simulink model "EDF2Tareas"  (R2021b)
settings: Solver=VariableStepAuto  StartTime=0.0  StopTime=0.2  RelTol=1e-3
values from neighbouring files (symbols this model uses):
  a = [8.878e-12  1.776e-11   2.663e-11]/0.0274    [GeneracionDatos.m]
  b = [1.291e-5   2.583e-5    3.874e-5]/0.0274    [GeneracionDatos.m]
  c = 0.0007648*[1 1 1]/0.0274    [GeneracionDatos.m]    (also in planner.m = zeros(N, 1))
  D = 0*[1 1 1]    [GeneracionDatos.m]
  H = H*gran    (= 0.001)    [GeneracionDatos.m]
  I = [5.1249     3.1462   1.4256]    [GeneracionDatos.m]
  N = length(h)    [GeneracionDatos.m]
  P = [0.028842   0.035017 0.039862]    [GeneracionDatos.m]
undefined symbols (not defined in the file or in its folder): m
libraries: slpidlib x3, sldelib x1
settings Model: Creator=YayoCG  LastModifiedBy=mluser
settings SolverCC: AlgebraicLoopSolver=TrustRegion
settings DebuggingCC: SFMachineParentedDataDiag=warning

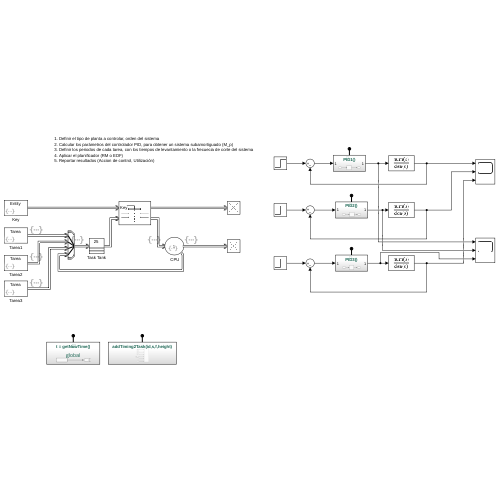
[thumbnail: Simulink's stored preview of the top-level diagram]
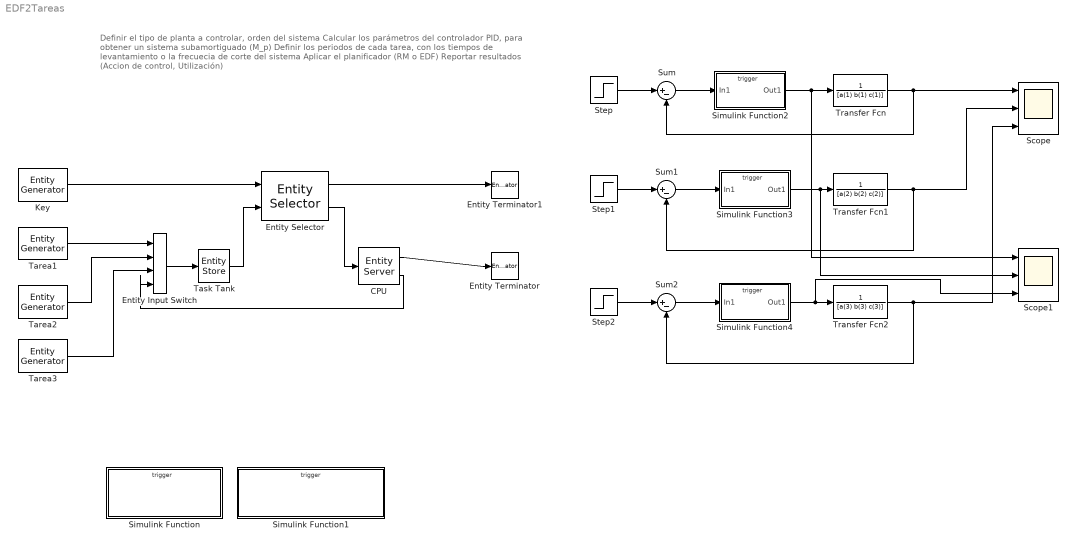
== system EDF2Tareas ==
  note: Definir el tipo de planta a controlar, orden del sistema
      | Calcular los parámetros del controlador PID, para obtener un sistema subamortiguado (M_p)
      | Definir los periodos de cada tarea, con los tiempos de levantamiento o la frecuecia de corte del sistema
      | Aplicar el planificador (RM o EDF)
      | Reportar resultados (Accion de control, Utilización)
  " CPU" : EntityServer  InputPortMessageModes=m  OutputPortMessageModes=m,m  Capacity=1  ServiceTimeSource=Attribute  ServiceTimeAttributeName=C  ServiceTimeAction=dt = entity.C + 0*rand(1,1);  EntryAction=|  ExitAction=|  PreemptAction=|  PermitPreemptionBasedOnAttribute=on  SortingAttributeName=C  WriteResidualTimeToAttribute=on  ResidualTimeAttributeName=C
      EntryAction=|
      | entity.priority = 2;
      | s = getNowTime();
      | entity.s = s;
      ExitAction=|
      | f = getNowTime();
      | addTiming2Task(entity.id, entity.s, f, 0.5);
      | 
      | switch entity.id
      |     case 1
      |         PID1();
      |     case 2
      |         PID2();
      |     case 3
      |         PID3();
      | end
      PreemptAction=|
      | %
      | f = getNowTime();
      | addTiming2Task(entity.id, entity.s, f, 0.5);
      settings: OutputPortMap=o9,o10
  Entity Input Switch : EntityInputSwitch  InputPortMessageModes=m,m,m,m  OutputPortMessageModes=m  NumberInputPorts=4
      settings: InputPortMap=u1,u2,u3,u4
  Entity Selector : sldelib/Entity Selector  mNumberOfStreams=1  mKeyEntityAttributeName={'key'}  mEntityAttributeName={'id'}  mMatchingNumberSource=Dialog  mNumberOfMatches=1  mNumberOfMatchesAttribute=Name  mNumEntitiesDepOpt=off  mNumEntitiesInBlockOpt=off  mNumEntitiesExtractedOpt=off
      settings: SourceProductBaseCode=SE
  Entity Terminator : EntityTerminator  InputPortMessageModes=m
  Entity Terminator1 : EntityTerminator  InputPortMessageModes=m
  Key : EntityGenerator  OutputPortMessageModes=m  TimeSource=MATLAB action  IntergenerationTimeAction=|  GenerateAction=|  AttributeName=key  AttributeInitialValue=0  EntityType=Structured  EntityTypeName=Entity
      IntergenerationTimeAction=|
      | persistent i;
      | 
      | if isempty(i)
      |     i = 0;
      | end
      | if i == length(Dt)
      |     i = 0;
      | end
      | 
      | i = i + 1;
      | dt = Dt(i);
      GenerateAction=|
      | persistent j;
      | 
      | if isempty(j)
      |     j = 0;
      | end
      | 
      | if j == length(idx)
      |     j = 0;      
      | end
      | 
      | j = j + 1;
      | entity.key = idx(j);
  Scope : Scope  NumInputPorts=3
  Scope1 : Scope  NumInputPorts=3
  Simulink Function : Subsystem  TreatAsAtomicUnit=on
  Simulink Function1 : Subsystem  TreatAsAtomicUnit=on
  Simulink Function2 : Subsystem  TreatAsAtomicUnit=on
  Simulink Function3 : Subsystem  TreatAsAtomicUnit=on
  Simulink Function4 : Subsystem  TreatAsAtomicUnit=on
  Step : Step  Time=0  SampleTime=0
  Step1 : Step  Time=0  SampleTime=0
  Step2 : Step  Time=0  SampleTime=0
  Sum : Sum  Inputs=|+-
  Sum1 : Sum  Inputs=|+-
  Sum2 : Sum  Inputs=|+-
  Tarea1 : EntityGenerator  OutputPortMessageModes=m  TimeSource=MATLAB action  IntergenerationTimeAction=dt = h(1) + 0*rand(1,1);  GenerateAction=|  ExitAction=|  AttributeName=h|C|s|priority|id  AttributeInitialValue=1|1|1|1|1  EntityType=Structured  EntityTypeName=Tarea
      GenerateAction=|
      | i = 1;
      | entity.id = i;
      | 
      | % entity.priority = selectTask(-1, i)
      | entity.h = h(i);
      | entity.C = C(i);
      ExitAction=|
      | f = getNowTime();
      | addTiming2Task(entity.id, f, f+1e-10, 1);
  Tarea2 : EntityGenerator  OutputPortMessageModes=m  TimeSource=MATLAB action  IntergenerationTimeAction=dt = h(2) + 0*rand(1,1);  GenerateAction=|  ExitAction=|  AttributeName=h|C|s|priority|id  AttributeInitialValue=1|1|1|1|1  EntityType=Structured  EntityTypeName=Tarea
      GenerateAction=|
      | i = 2;
      | entity.id = i;
      | 
      | % entity.priority = selectTask(-1, i)
      | entity.h = h(i);
      | entity.C = C(i);
      ExitAction=|
      | f = getNowTime();
      | addTiming2Task(entity.id, f, f+1e-10, 1);
  Tarea3 : EntityGenerator  OutputPortMessageModes=m  TimeSource=MATLAB action  IntergenerationTimeAction=dt = h(3) + 0*rand(1,1);  GenerateAction=|  ExitAction=|  AttributeName=h|C|s|priority|id  AttributeInitialValue=1|1|1|1|1  EntityType=Structured  EntityTypeName=Tarea
      GenerateAction=|
      | i = 3;
      | entity.id = i;
      | 
      | % entity.priority = selectTask(-1, i)
      | entity.h = h(i);
      | entity.C = C(i);
      ExitAction=|
      | f = getNowTime();
      | addTiming2Task(entity.id, f, f+1e-10, 1);
  Task Tank : EntityStore  InputPortMessageModes=m  OutputPortMessageModes=m  EntryAction=entity.priority = 1;
      settings: OutputPortMap=o4
  Transfer Fcn : TransferFcn  Denominator=[a(1) b(1) c(1)]
  Transfer Fcn1 : TransferFcn  Denominator=[a(2) b(2) c(2)]
  Transfer Fcn2 : TransferFcn  Denominator=[a(3) b(3) c(3)]
  wires:
  Tarea1/1 -> Entity Input Switch/1
  Tarea2/1 -> Entity Input Switch/2
  Tarea3/1 -> Entity Input Switch/3
  Step/1 -> Sum/1
  Transfer Fcn/1 -> Scope/1, Sum/2
  Transfer Fcn1/1 -> Scope/2, Sum1/2
  Step1/1 -> Sum1/1
  Step2/1 -> Sum2/1
  Transfer Fcn2/1 -> Sum2/2, Scope/3
  Sum/1 -> Simulink Function2/1(In1)
  Sum1/1 -> Simulink Function3/1(In1)
  Sum2/1 -> Simulink Function4/1(In1)
  Simulink Function2/1(Out1) -> Scope1/1, Transfer Fcn/1
  Simulink Function3/1(Out1) -> Scope1/2, Transfer Fcn1/1
  Simulink Function4/1(Out1) -> Scope1/3, Transfer Fcn2/1
  Entity Selector/2 -> " CPU"/1
  " CPU"/1 -> Entity Terminator/1
  " CPU"/2 -> Entity Input Switch/4
  Entity Selector/1 -> Entity Terminator1/1
  Entity Input Switch/1 -> Task Tank/1
  Task Tank/1 -> Entity Selector/2
  Key/1 -> Entity Selector/1

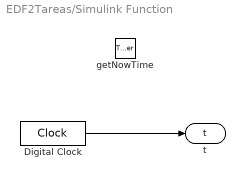
== system EDF2Tareas/Simulink Function ==
  getNowTime : TriggerPort  TriggerType=function-call  IsSimulinkFunction=on  FunctionName=getNowTime  VariantControl=(inherit)
  Digital Clock : DigitalClock  SampleTime=-1
  t : ArgOut  DisableCoverage=on  ArgumentName=t
  wires:
  Digital Clock/1 -> t/1

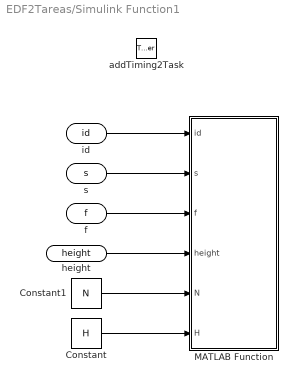
== system EDF2Tareas/Simulink Function1 ==
  addTiming2Task : TriggerPort  TriggerType=function-call  IsSimulinkFunction=on  FunctionName=addTiming2Task  FunctionVisibility=scoped  VariantControl=(inherit)
  Constant : Constant  Value=H
  Constant1 : Constant  Value=N
  MATLAB Function : MATLAB Function  TreatAsAtomicUnit=on
  id : ArgIn  DisableCoverage=on  ArgumentName=id
  s : ArgIn  DisableCoverage=on  Port=2  ArgumentName=s
  f : ArgIn  DisableCoverage=on  Port=3  ArgumentName=f
  height : ArgIn  DisableCoverage=on  Port=4  ArgumentName=height
  wires:
  id/1 -> MATLAB Function/1(id)
  s/1 -> MATLAB Function/2(s)
  f/1 -> MATLAB Function/3(f)
  Constant/1 -> MATLAB Function/6(H)
  height/1 -> MATLAB Function/4(height)
  Constant1/1 -> MATLAB Function/5(N)

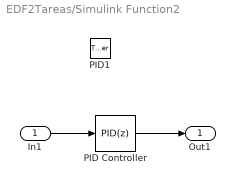
== system EDF2Tareas/Simulink Function2 ==
  In1 : Inport
  PID1 : TriggerPort  TriggerType=function-call  IsSimulinkFunction=on  FunctionName=PID1  FunctionVisibility=scoped  VariantControl=(inherit)
  PID Controller : slpidlib/PID Controller  Controller=PID  Form=Parallel  TimeDomain=Discrete-time  UseExternalTs=off  SampleTime=-1  IntegratorMethod=Forward Euler  FilterMethod=Forward Euler  ControllerParametersSource=internal  P=P(1)  I=I(1)  D=D(1)  UseFilter=on  N=100  TunerSelectOption=Frequency Response Based  InitialConditionSource=internal  InitialConditionForIntegrator=0  InitialConditionForFilter=0  DifferentiatorICPrevScaledInput=0  ExternalReset=none  TrackingMode=off  Kt=1  LimitOutput=off  SatLimitsSource=internal  UpperSaturationLimit=inf  LowerSaturationLimit=-inf  LinearizeAsGain=on  AntiWindupMode=none  Kb=1  POutMin=[]  POutMax=[]  IOutMin=[]  IOutMax=[]  DOutMin=[]  DOutMax=[]  NOutMin=[]  NOutMax=[]  SumOutMin=[]  SumOutMax=[]  SaturationOutMin=[]  SaturationOutMax=[]  PParamMin=[]  PParamMax=[]  IParamMin=[]  IParamMax=[]  DParamMin=[]  DParamMax=[]  NParamMin=[]  NParamMax=[]  KbParamMin=[]  KbParamMax=[]  KtParamMin=[]  KtParamMax=[]  KbOutMin=[]  KbOutMax=[]  KtOutMin=[]  KtOutMax=[]  IntegratorOutMin=[]  IntegratorOutMax=[]  FilterOutMin=[]  FilterOutMax=[]  SumI1OutMin=[]  SumI1OutMax=[]  SumI2OutMin=[]  SumI2OutMax=[]  SumI3OutMin=[]  SumI3OutMax=[]  SumI4OutMin=[]  SumI4OutMax=[]  SumDOutMin=[]  SumDOutMax=[]  DifferentiatorOutMin=[]  DifferentiatorOutMax=[]  FilterDiffOutCoefMin=[]  FilterDiffOutCoefMax=[]  ReciprocalOutMin=[]  ReciprocalOutMax=[]  SumDenOutMin=[]  SumDenOutMax=[]  SumNumOutMin=[]  SumNumOutMax=[]  DivideOutMin=[]  DivideOutMax=[]  UdiffTsProdOutMin=[]  UdiffTsProdOutMax=[]  NTsProdOutMin=[]  NTsProdOutMax=[]  UintegralTsProdOutMin=[]  UintegralTsProdOutMax=[]  UngainTsProdOutMin=[]  UngainTsProdOutMax=[]  IntegratorContinuousStateAttributes=''  IntegratorStateMustResolveToSignalObject=off  IntegratorRTWStateStorageClass=Auto  FilterContinuousStateAttributes=''  FilterStateMustResolveToSignalObject=off  FilterRTWStateStorageClass=Auto  ParallelPVariant=InternalParameters  IdealPVariant=Disabled  IVariant=InternalParameters  DVariant=InternalParameters  IntegratorVariant=Discrete  SatVariant=Disabled  AWVariant=Passthrough  PCopyVariant=Disabled  TRVariant=Disabled  FdbkBlocksVariant=Forward  IdealPFdbkVariant=Disabled  SatFdbkVariant=Disabled  DerivativeFilterVariant=ForwardEulerFilter  NVariant=InternalParameters  NCopyVariant=Disabled  FilterICVariant=InternalICsFilter  IntegratorICVariant=InternalICs  ExternalResetVariant=Disabled  TRSumVariant=Passthrough  SumFdbkVariant=Disabled  SumVariant=Sum_PID  TsampFilterVariant=InternalTs  TsampNgainVariant=Passthrough  TsampIntegralVariant=Passthrough  ExternalSaturationOutDataTypeStr=Inherit: Same as second input
  Out1 : Outport
  wires:
  In1/1 -> PID Controller/1
  PID Controller/1 -> Out1/1

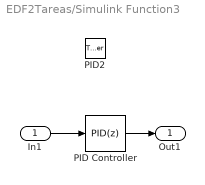
== system EDF2Tareas/Simulink Function3 ==
  In1 : Inport
  PID2 : TriggerPort  TriggerType=function-call  IsSimulinkFunction=on  FunctionName=PID2  FunctionVisibility=scoped  VariantControl=(inherit)
  PID Controller : slpidlib/PID Controller  Controller=PID  Form=Parallel  TimeDomain=Discrete-time  UseExternalTs=off  SampleTime=-1  IntegratorMethod=Forward Euler  FilterMethod=Forward Euler  ControllerParametersSource=internal  P=P(2)  I=I(2)  D=D(2)  UseFilter=on  N=100  TunerSelectOption=Frequency Response Based  InitialConditionSource=internal  InitialConditionForIntegrator=0  InitialConditionForFilter=0  DifferentiatorICPrevScaledInput=0  ExternalReset=none  TrackingMode=off  Kt=1  LimitOutput=off  SatLimitsSource=internal  UpperSaturationLimit=inf  LowerSaturationLimit=-inf  LinearizeAsGain=on  AntiWindupMode=none  Kb=1  POutMin=[]  POutMax=[]  IOutMin=[]  IOutMax=[]  DOutMin=[]  DOutMax=[]  NOutMin=[]  NOutMax=[]  SumOutMin=[]  SumOutMax=[]  SaturationOutMin=[]  SaturationOutMax=[]  PParamMin=[]  PParamMax=[]  IParamMin=[]  IParamMax=[]  DParamMin=[]  DParamMax=[]  NParamMin=[]  NParamMax=[]  KbParamMin=[]  KbParamMax=[]  KtParamMin=[]  KtParamMax=[]  KbOutMin=[]  KbOutMax=[]  KtOutMin=[]  KtOutMax=[]  IntegratorOutMin=[]  IntegratorOutMax=[]  FilterOutMin=[]  FilterOutMax=[]  SumI1OutMin=[]  SumI1OutMax=[]  SumI2OutMin=[]  SumI2OutMax=[]  SumI3OutMin=[]  SumI3OutMax=[]  SumI4OutMin=[]  SumI4OutMax=[]  SumDOutMin=[]  SumDOutMax=[]  DifferentiatorOutMin=[]  DifferentiatorOutMax=[]  FilterDiffOutCoefMin=[]  FilterDiffOutCoefMax=[]  ReciprocalOutMin=[]  ReciprocalOutMax=[]  SumDenOutMin=[]  SumDenOutMax=[]  SumNumOutMin=[]  SumNumOutMax=[]  DivideOutMin=[]  DivideOutMax=[]  UdiffTsProdOutMin=[]  UdiffTsProdOutMax=[]  NTsProdOutMin=[]  NTsProdOutMax=[]  UintegralTsProdOutMin=[]  UintegralTsProdOutMax=[]  UngainTsProdOutMin=[]  UngainTsProdOutMax=[]  IntegratorContinuousStateAttributes=''  IntegratorStateMustResolveToSignalObject=off  IntegratorRTWStateStorageClass=Auto  FilterContinuousStateAttributes=''  FilterStateMustResolveToSignalObject=off  FilterRTWStateStorageClass=Auto  ParallelPVariant=InternalParameters  IdealPVariant=Disabled  IVariant=InternalParameters  DVariant=InternalParameters  IntegratorVariant=Discrete  SatVariant=Disabled  AWVariant=Passthrough  PCopyVariant=Disabled  TRVariant=Disabled  FdbkBlocksVariant=Forward  IdealPFdbkVariant=Disabled  SatFdbkVariant=Disabled  DerivativeFilterVariant=ForwardEulerFilter  NVariant=InternalParameters  NCopyVariant=Disabled  FilterICVariant=InternalICsFilter  IntegratorICVariant=InternalICs  ExternalResetVariant=Disabled  TRSumVariant=Passthrough  SumFdbkVariant=Disabled  SumVariant=Sum_PID  TsampFilterVariant=InternalTs  TsampNgainVariant=Passthrough  TsampIntegralVariant=Passthrough  ExternalSaturationOutDataTypeStr=Inherit: Same as second input
  Out1 : Outport
  wires:
  PID Controller/1 -> Out1/1
  In1/1 -> PID Controller/1

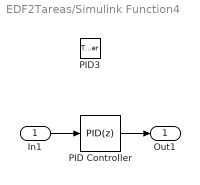
== system EDF2Tareas/Simulink Function4 ==
  In1 : Inport
  PID3 : TriggerPort  TriggerType=function-call  IsSimulinkFunction=on  FunctionName=PID3  FunctionVisibility=scoped  VariantControl=(inherit)
  PID Controller : slpidlib/PID Controller  Controller=PID  Form=Parallel  TimeDomain=Discrete-time  UseExternalTs=off  SampleTime=-1  IntegratorMethod=Forward Euler  FilterMethod=Forward Euler  ControllerParametersSource=internal  P=P(3)  I=I(3)  D=D(3)  UseFilter=on  N=100  TunerSelectOption=Frequency Response Based  InitialConditionSource=internal  InitialConditionForIntegrator=0  InitialConditionForFilter=0  DifferentiatorICPrevScaledInput=0  ExternalReset=none  TrackingMode=off  Kt=1  LimitOutput=off  SatLimitsSource=internal  UpperSaturationLimit=inf  LowerSaturationLimit=-inf  LinearizeAsGain=on  AntiWindupMode=none  Kb=1  POutMin=[]  POutMax=[]  IOutMin=[]  IOutMax=[]  DOutMin=[]  DOutMax=[]  NOutMin=[]  NOutMax=[]  SumOutMin=[]  SumOutMax=[]  SaturationOutMin=[]  SaturationOutMax=[]  PParamMin=[]  PParamMax=[]  IParamMin=[]  IParamMax=[]  DParamMin=[]  DParamMax=[]  NParamMin=[]  NParamMax=[]  KbParamMin=[]  KbParamMax=[]  KtParamMin=[]  KtParamMax=[]  KbOutMin=[]  KbOutMax=[]  KtOutMin=[]  KtOutMax=[]  IntegratorOutMin=[]  IntegratorOutMax=[]  FilterOutMin=[]  FilterOutMax=[]  SumI1OutMin=[]  SumI1OutMax=[]  SumI2OutMin=[]  SumI2OutMax=[]  SumI3OutMin=[]  SumI3OutMax=[]  SumI4OutMin=[]  SumI4OutMax=[]  SumDOutMin=[]  SumDOutMax=[]  DifferentiatorOutMin=[]  DifferentiatorOutMax=[]  FilterDiffOutCoefMin=[]  FilterDiffOutCoefMax=[]  ReciprocalOutMin=[]  ReciprocalOutMax=[]  SumDenOutMin=[]  SumDenOutMax=[]  SumNumOutMin=[]  SumNumOutMax=[]  DivideOutMin=[]  DivideOutMax=[]  UdiffTsProdOutMin=[]  UdiffTsProdOutMax=[]  NTsProdOutMin=[]  NTsProdOutMax=[]  UintegralTsProdOutMin=[]  UintegralTsProdOutMax=[]  UngainTsProdOutMin=[]  UngainTsProdOutMax=[]  IntegratorContinuousStateAttributes=''  IntegratorStateMustResolveToSignalObject=off  IntegratorRTWStateStorageClass=Auto  FilterContinuousStateAttributes=''  FilterStateMustResolveToSignalObject=off  FilterRTWStateStorageClass=Auto  ParallelPVariant=InternalParameters  IdealPVariant=Disabled  IVariant=InternalParameters  DVariant=InternalParameters  IntegratorVariant=Discrete  SatVariant=Disabled  AWVariant=Passthrough  PCopyVariant=Disabled  TRVariant=Disabled  FdbkBlocksVariant=Forward  IdealPFdbkVariant=Disabled  SatFdbkVariant=Disabled  DerivativeFilterVariant=ForwardEulerFilter  NVariant=InternalParameters  NCopyVariant=Disabled  FilterICVariant=InternalICsFilter  IntegratorICVariant=InternalICs  ExternalResetVariant=Disabled  TRSumVariant=Passthrough  SumFdbkVariant=Disabled  SumVariant=Sum_PID  TsampFilterVariant=InternalTs  TsampNgainVariant=Passthrough  TsampIntegralVariant=Passthrough  ExternalSaturationOutDataTypeStr=Inherit: Same as second input
  Out1 : Outport
  wires:
  In1/1 -> PID Controller/1
  PID Controller/1 -> Out1/1

== matlab function EDF2Tareas/Simulink Function1/MATLAB Function ==
  data: id input; s input; f input; height input; N input; H input
function fcn(id, s, f, height, N, H)    
      
    persistent ax 

    cBlue = [18/255 104/255 179/255];
    cRed = [237/255 36/255 38/255];
    cGreen = [155 190 61]/255;
    allColors = [cBlue; cRed; cGreen];

    if isempty(ax)
        close all;
        fig = figure('position',[762 173 920 326]);
        ax = axes;
        set(ax,'box','on');
        grid on; hold on;
        set(ax,'XLim',[0 H],'YLim',[1 N+1],'YTick',1:N+1,'xminorgrid','on');
        set(fig,'name','Task Timing');

    end

    rectangle('parent', ax, ...
              'position', [s, id, f-s, height], ...
              'facecolor', allColors(id,:));

end
